simulink model "regolatore"  (R2020b)
settings: Solver=VariableStepAuto  StartTime=0.0  StopTime=5  MaxStep=1e-3  RelTol=1e-3
values from neighbouring files (symbols this model uses):
  A = [ 0 1; 900 0]    [regolatore_16_04.m]
  alpha = 1    [regolatore_16_04.m]
  B = [ 0 -9]'    [regolatore_16_04.m]
  C = [ 600 0]    [regolatore_16_04.m]
  K = place(A, B, auto_des_controllo)    [regolatore_16_04.m]
  L = Lt'    [regolatore_16_04.m]
settings Model: Creator=serra  LastModifiedBy=serra

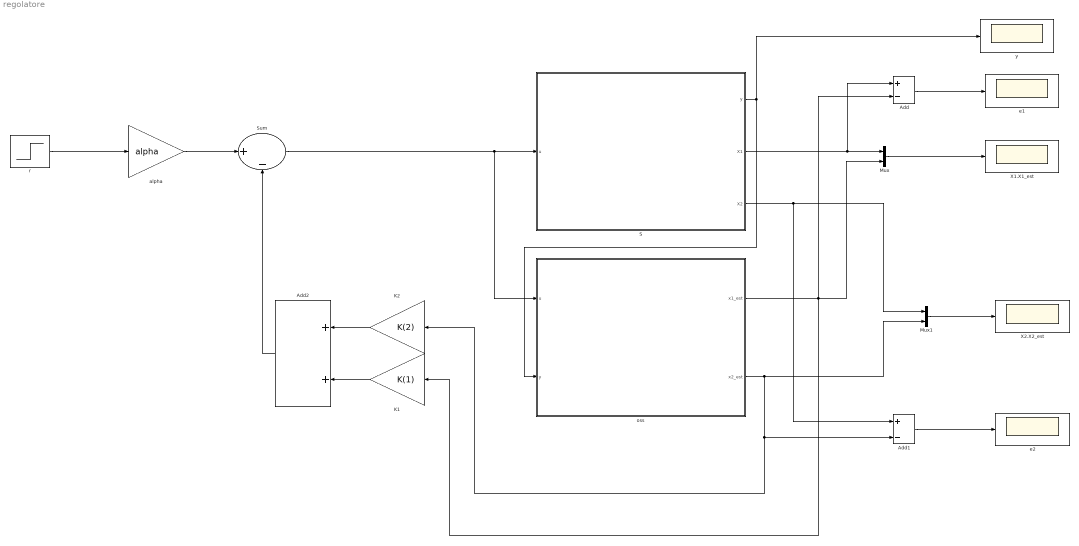
== system regolatore ==
  Add : Sum  Inputs=+-
  Add1 : Sum  Inputs=+-
  Add2 : Sum
  K1 : Gain  Gain=K(1)
  K2 : Gain  Gain=K(2)
  Mux : Mux  Inputs=2
  Mux1 : Mux  Inputs=2
  S : Subsystem
  Sum : Sum  Inputs=|+-
  X1.X1_est : Scope
  X2.X2_est : Scope
  alpha : Gain  Gain=alpha
  e1 : Scope
  e2 : Scope
  oss : Subsystem
  r : Step  Time=0  SampleTime=0
  y : Scope
  wires:
  oss/2(x2_est) -> K2/1, Add1/2, Mux1/2
  S/1(y) -> y/1, oss/2(y)
  Add/1 -> e1/1
  Mux/1 -> X1.X1_est/1
  Mux1/1 -> X2.X2_est/1
  Add1/1 -> e2/1
  S/3(X2) -> Add1/1, Mux1/1
  oss/1(x1_est) -> K1/1, Add/2, Mux/2
  S/2(X1) -> Add/1, Mux/1
  r/1 -> alpha/1
  alpha/1 -> Sum/1
  Add2/1 -> Sum/2
  K2/1 -> Add2/1
  K1/1 -> Add2/2
  Sum/1 -> oss/1(u), S/1(u)

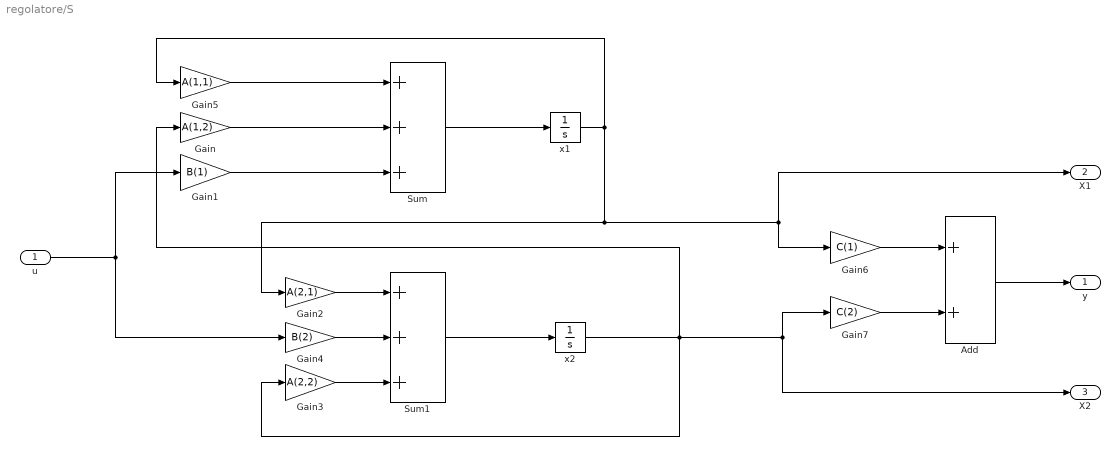
== system regolatore/S ==
  u : Inport
  Add : Sum
  Gain : Gain  Gain=A(1,2)
  Gain1 : Gain  Gain=B(1)
  Gain2 : Gain  Gain=A(2,1)
  Gain3 : Gain  Gain=A(2,2)
  Gain4 : Gain  Gain=B(2)
  Gain5 : Gain  Gain=A(1,1)
  Gain6 : Gain  Gain=C(1)
  Gain7 : Gain  Gain=C(2)
  Sum : Sum  Inputs=+++
  Sum1 : Sum  Inputs=+++
  x1 : Integrator  InitialCondition=-5
  x2 : Integrator  InitialCondition=1
  y : Outport
  X1 : Outport  Port=2
  X2 : Outport  Port=3
  wires:
  Sum1/1 -> x2/1
  Add/1 -> y/1
  Gain1/1 -> Sum/3
  Sum/1 -> x1/1
  Gain2/1 -> Sum1/1
  x2/1 -> Gain3/1, Gain/1, Gain7/1, X2/1
  Gain/1 -> Sum/2
  Gain3/1 -> Sum1/3
  Gain4/1 -> Sum1/2
  u/1 -> Gain4/1, Gain1/1
  x1/1 -> Gain5/1, Gain2/1, X1/1, Gain6/1
  Gain5/1 -> Sum/1
  Gain6/1 -> Add/1
  Gain7/1 -> Add/2

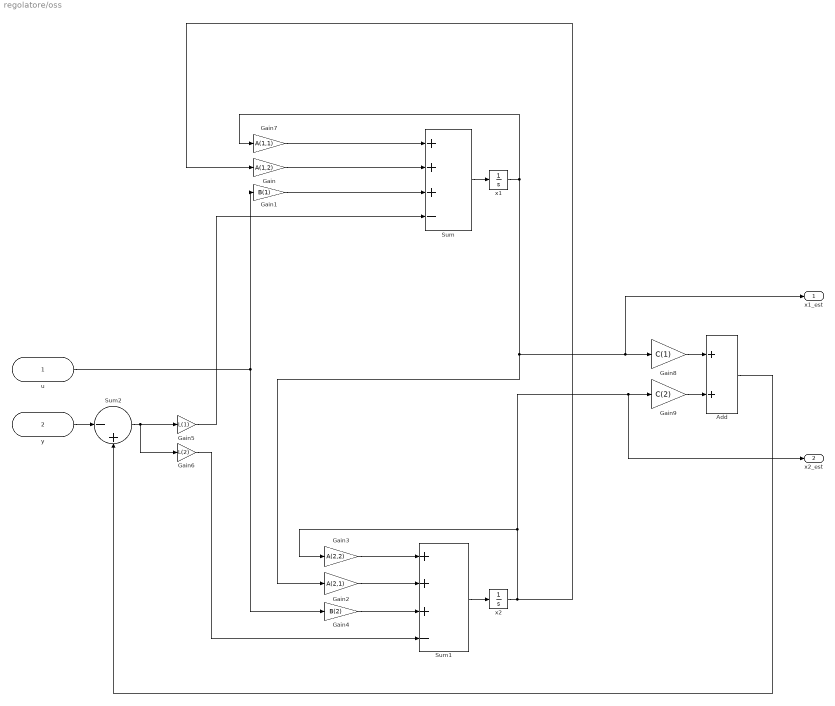
== system regolatore/oss ==
  u : Inport
  y : Inport  Port=2
  Add : Sum
  Gain : Gain  Gain=A(1,2)
  Gain1 : Gain  Gain=B(1)
  Gain2 : Gain  Gain=A(2,1)
  Gain3 : Gain  Gain=A(2,2)
  Gain4 : Gain  Gain=B(2)
  Gain5 : Gain  Gain=L(1)
  Gain6 : Gain  Gain=L(2)
  Gain7 : Gain  Gain=A(1,1)
  Gain8 : Gain  Gain=C(1)
  Gain9 : Gain  Gain=C(2)
  Sum : Sum  Inputs=+++-
  Sum1 : Sum  Inputs=+++-
  Sum2 : Sum  Inputs=|-+
  x1 : Integrator
  x2 : Integrator
  x1_est : Outport
  x2_est : Outport  Port=2
  wires:
  Sum1/1 -> x2/1
  Gain/1 -> Sum/2
  Add/1 -> Sum2/2
  x1/1 -> x1_est/1, Gain8/1, Gain2/1, Gain7/1
  Gain1/1 -> Sum/3
  Sum/1 -> x1/1
  x2/1 -> Gain/1, x2_est/1, Gain9/1, Gain3/1
  u/1 -> Gain4/1, Gain1/1
  Gain4/1 -> Sum1/3
  y/1 -> Sum2/1
  Sum2/1 -> Gain6/1, Gain5/1
  Gain5/1 -> Sum/4
  Gain6/1 -> Sum1/4
  Gain7/1 -> Sum/1
  Gain3/1 -> Sum1/1
  Gain2/1 -> Sum1/2
  Gain9/1 -> Add/2
  Gain8/1 -> Add/1
